simulink library "FlatSatWrite_lib"  (R2018b)
settings: Solver=VariableStepAuto  StartTime=0.0  StopTime=10.0  RelTol=1e-3
settings Model: Creator=Taylor  LastModifiedBy=Taylor

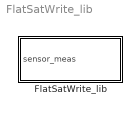
== system FlatSatWrite_lib ==
  FlatSatWrite_lib : Subsystem

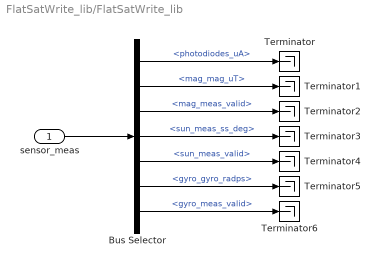
== system FlatSatWrite_lib/FlatSatWrite_lib ==
  sensor_meas : Inport  OutDataTypeStr=Bus: sensor_bus
  Bus Selector : BusSelector  OutputSignals=photodiodes_uA,mag_mag_uT,mag_meas_valid,sun_meas_ss_deg,sun_meas_valid,gyro_gyro_radps,gyro_meas_valid
  Terminator{,1..6} (7 alike) : Terminator
  wires:
  sensor_meas/1 -> Bus Selector/1
  Bus Selector/1 -> Terminator/1  "<photodiodes_uA>"
  Bus Selector/2 -> Terminator1/1  "<mag_mag_uT>"
  Bus Selector/3 -> Terminator2/1  "<mag_meas_valid>"
  Bus Selector/4 -> Terminator3/1  "<sun_meas_ss_deg>"
  Bus Selector/5 -> Terminator4/1  "<sun_meas_valid>"
  Bus Selector/6 -> Terminator5/1  "<gyro_gyro_radps>"
  Bus Selector/7 -> Terminator6/1  "<gyro_meas_valid>"
